simulink model "qusetion1_1"  (R2016b)
settings: Solver=VariableStepAuto  StartTime=0.0  StopTime=10.0  RelTol=1e-3
settings Model: Creator=dell  LastModifiedBy=dell

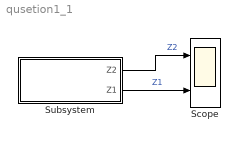
== system qusetion1_1 ==
  Scope : Scope  NumInputPorts=2
  Subsystem : Subsystem  mask{A=0, B=0, C=0}
  wires:
  Subsystem/1(Z2) -> Scope/1  "Z2"
  Subsystem/2(Z1) -> Scope/2  "Z1"

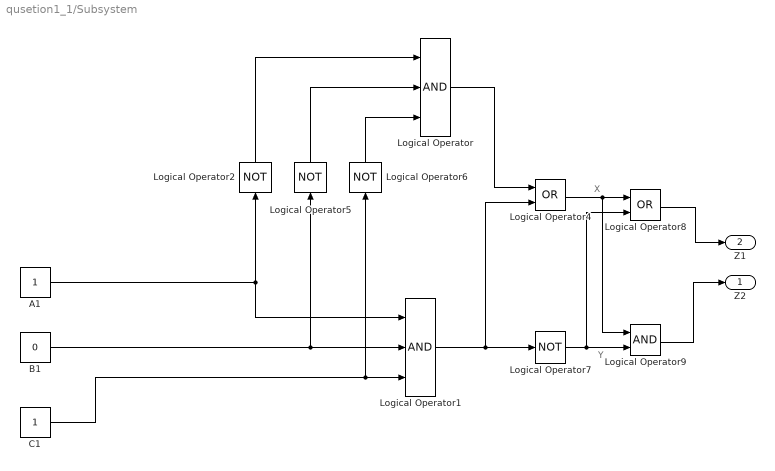
== system qusetion1_1/Subsystem ==
  note: Y
  note: X
  A1 : Constant
  B1 : Constant  Value=0
  C1 : Constant
  Logical Operator : Logic  Inputs=3  AllPortsSameDT=off  OutDataTypeStr=boolean
  Logical Operator1 : Logic  Inputs=3  AllPortsSameDT=off  OutDataTypeStr=boolean
  Logical Operator{2,5..7} (4 alike) : Logic  Operator=NOT  AllPortsSameDT=off  OutDataTypeStr=boolean
  Logical Operator4 : Logic  Operator=OR  AllPortsSameDT=off  OutDataTypeStr=boolean
  Logical Operator8 : Logic  Operator=OR  AllPortsSameDT=off  OutDataTypeStr=boolean
  Logical Operator9 : Logic  AllPortsSameDT=off  OutDataTypeStr=boolean
  Z2 : Outport
  Z1 : Outport  Port=2
  wires:
  Logical Operator/1 -> Logical Operator4/1
  Logical Operator6/1 -> Logical Operator/3
  Logical Operator5/1 -> Logical Operator/2
  Logical Operator2/1 -> Logical Operator/1
  A1/1 -> Logical Operator1/1, Logical Operator2/1
  C1/1 -> Logical Operator6/1, Logical Operator1/3
  Logical Operator1/1 -> Logical Operator4/2, Logical Operator7/1
  B1/1 -> Logical Operator5/1, Logical Operator1/2
  Logical Operator4/1 -> Logical Operator9/1, Logical Operator8/1
  Logical Operator7/1 -> Logical Operator8/2, Logical Operator9/2
  Logical Operator9/1 -> Z2/1
  Logical Operator8/1 -> Z1/1
